simulink subsystem "AS_ExhalationCircuit"  (R2022b)
settings: Solver=VariableStepAuto  StartTime=0.0  StopTime=10.0  RelTol=1e-3
undefined symbols (not defined in the file): cmH2O_to_Pa, Exhalation_Opening_Height, Exhalation_Restrict_Dia, PIDiameter
libraries: fl_lib x6, nesl_utility x3, SimscapeFluids_lib x1
settings Model: DefaultTestHarness=AS_ExhalationCircuit_Harness  Creator=CSN-Simulation  LastModifiedBy=MATLAB
settings DebuggingCC: UnconnectedInputMsg=warning  UnconnectedOutputMsg=warning  UnconnectedLineMsg=warning
settings ModelReferenceCC: EnableRefExpFcnMdlSchedulingChecks=on
settings RTWCC: DLArmComputeVersion=19.05

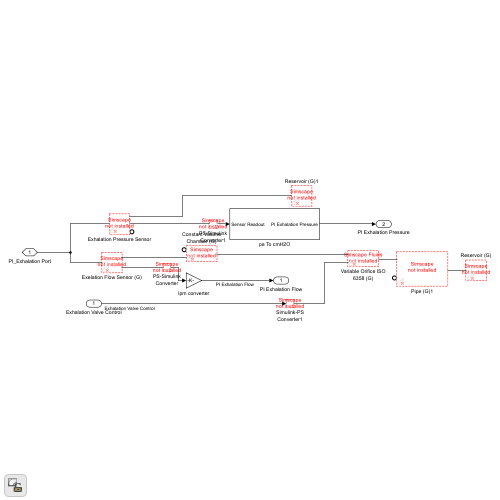
[thumbnail: Simulink's stored preview of the top-level diagram]
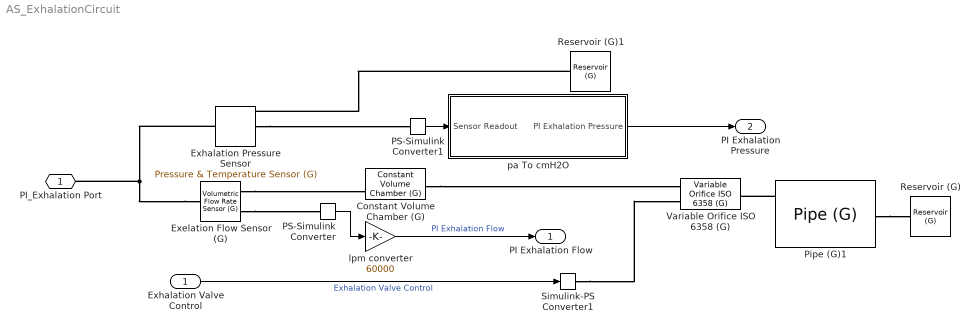
== system AS_ExhalationCircuit ==
  Exhalation Valve Control : Inport
  Constant Volume Chamber (G) : fl_lib/Gas/Elements/Constant Volume Chamber (G)  volume=12000 mm^3  num_ports=foundation.enum.num_ports.two  area_A=pi*(PIDiameter/2)^2 mm^2  area_B=pi*Exhalation_Restrict_Dia*Exhalation_Opening_Height+1 mm^2  area_C=0.01 m^2  area_D=0.01 m^2  p_I_specify=off  p_I_priority=High  p_I=0.101325 MPa  p_I_nominal_specify=off  p_I_nominal_unit=MPa  p_I_nominal_value=1  T_I_specify=off  T_I_priority=High  T_I=293.15 K  T_I_nominal_specify=off  T_I_nominal_unit=K  T_I_nominal_value=1  rho_chamber_specify=off  rho_chamber_priority=None  rho_chamber=1.2 kg/m^3  rho_chamber_nominal_specify=off  rho_chamber_nominal_unit=kg/m^3  rho_chamber_nominal_value=1
      settings: InternalSimscapePortConfiguration="{\"Bottom\":[],\"Left\":[{\"id\":\"A\",\"label\":\"A\",\"type\":\"foundation.gas.gas\"},{\"id\":\"H\",\"label\":\"H\",\"type\":\"foundation.thermal.thermal\"}],\"Right\":[{\"id\":\"B\",\"label\":\"B\",\"type\":\"foundation.gas.gas\"}],\"Top\":[]}"
  Exelation Flow Sensor (G) : fl_lib/Gas/Sensors/Volumetric Flow Rate Sensor (G)
      settings: InternalSimscapePortConfiguration="{\"Bottom\":[],\"Left\":[{\"id\":\"A\",\"label\":\"A\",\"type\":\"foundation.gas.gas\"}],\"Right\":[{\"id\":\"B\",\"label\":\"B\",\"type\":\"foundation.gas.gas\"},{\"id\":\"V\",\"label\":\"V\",\"type\":\"output\"}],\"Top\":[]}"
  Exhalation Pressure Sensor : fl_lib/Gas/Sensors/Pressure & Temperature Sensor (G)
      settings: InternalSimscapePortConfiguration="{\"Bottom\":[],\"Left\":[{\"id\":\"A\",\"label\":\"A\",\"type\":\"foundation.gas.gas\"}],\"Right\":[{\"id\":\"B\",\"label\":\"B\",\"type\":\"foundation.gas.gas\"},{\"id\":\"P\",\"label\":\"P\",\"type\":\"output\"},{\"id\":\"T\",\"label\":\"T\",\"type\":\"output\"}],\"Top\":[]}"
  PS-Simulink Converter : nesl_utility/PS-Simulink Converter  PhysicalDomain=network_engine_domain  SubClassName=ps_output  LeftPortType=input  RightPortType=output  PseudoPeriodic=off  Frequencies=[]  Unit=inherit  AffineConversion=off
  PS-Simulink Converter1 : nesl_utility/PS-Simulink Converter  PhysicalDomain=network_engine_domain  SubClassName=ps_output  LeftPortType=input  RightPortType=output  PseudoPeriodic=off  Frequencies=[]  Unit=inherit  AffineConversion=off
  Pipe (G)1 : fl_lib/Gas/Elements/Pipe (G)  length=5 mm  area=pi*Exhalation_Restrict_Dia*Exhalation_Opening_Height+1 mm^2  Dh=PIDiameter mm  length_add=0.1 m  roughness=15e-6 m  Re_lam=2000  Re_tur=4000  shape_factor=64  Nu_lam=3.66  p_I_specify=off  p_I_priority=High  p_I=0.101325 MPa  p_I_nominal_specify=off  p_I_nominal_unit=MPa  p_I_nominal_value=1  T_I_specify=on  T_I_priority=High  T_I=T_room degC  T_I_nominal_specify=off  T_I_nominal_unit=K  T_I_nominal_value=1  rho_pipe_specify=off  rho_pipe_priority=None  rho_pipe=1.2 kg/m^3  rho_pipe_nominal_specify=off  rho_pipe_nominal_unit=kg/m^3  rho_pipe_nominal_value=1
  Reservoir (G) : fl_lib/Gas/Elements/Reservoir (G)  pressure_spec=foundation.enum.pressure_spec.atmospheric  reservoir_pressure=0.101325 MPa  reservoir_temperature=T_room degC  area_A=pi*(PIDiameter/2)^2 mm^2
  Reservoir (G)1 : fl_lib/Gas/Elements/Reservoir (G)  pressure_spec=foundation.enum.pressure_spec.atmospheric  reservoir_pressure=0.101325 MPa  reservoir_temperature=293.15 K  area_A=0.01 m^2
  Simulink-PS Converter1 : nesl_utility/Simulink-PS Converter  PhysicalDomain=network_engine_domain  SubClassName=ps_input  LeftPortType=input  RightPortType=output  PseudoPeriodic=off  Frequencies=[]  NoiseDistribution=none  NoiseParameters=[]  Unit=1  AffineConversion=off  FilteringAndDerivatives=provide  SimscapeFilterOrder=1  InputFilterTimeConstant=0.001  UdotUserProvided=0
  Variable Orifice ISO 6358 (G) : SimscapeFluids_lib/Gas/Valves & Orifices/Variable Orifice ISO 6358 (G)  iso_cond_spec=fluids.gas.enum.iso_cond_spec.area  iso_opening_spec_C=fluids.gas.enum.iso_opening_spec.linear  C_max=1.6 l/s/bar  C_min=1e-5 l/s/bar  B_crit=0.3  opening_C_TLU=0 : 0.2 : 1  C_TLU=[1e-05, .32, .64, .96, 1.28, 1.6] l/s/bar  B_crit_TLU=0.3 * ones(1, 6)  m=0.5  iso_opening_spec_Cv=fluids.gas.enum.iso_opening_spec.linear  Cv_max=0.4  Cv_min=1e-6  opening_Cv_TLU=0 : 0.2 : 1  Cv_TLU=[1e-06, .08, .16, .24, .32, .4]  iso_opening_spec_Kv=fluids.gas.enum.iso_opening_spec.linear  Kv_max=0.3  Kv_min=1e-6  opening_Kv_TLU=0 : 0.2 : 1  Kv_TLU=[1e-06, .06, .12, .18, .24, .3]  iso_opening_spec_area=fluids.gas.enum.iso_opening_spec.linear  restriction_area_max=pi*Exhalation_Restrict_Dia*Exhalation_Opening_Height mm^2  restriction_area_min=1e-10 mm^2  opening_area_TLU=0 : 0.2 : 1  restriction_area_TLU=[1e-10, 2e-06, 4e-06, 6e-06, 8e-06, 1e-05] m^2  area=pi*Exhalation_Restrict_Dia*Exhalation_Opening_Height+1 mm^2  B_lam=0.999  T0=293.15 K  rho0=1.185 kg/m^3  smoothing_factor=0
      settings: InternalSimscapePortConfiguration="{\"Bottom\":[],\"Left\":[{\"id\":\"A\",\"label\":\"A\",\"type\":\"foundation.gas.gas\"},{\"id\":\"L\",\"label\":\"L\",\"type\":\"input\"}],\"Right\":[{\"id\":\"B\",\"label\":\"B\",\"type\":\"foundation.gas.gas\"}],\"Top\":[]}"
  lpm converter : Gain  Gain=60000
  pa To cmH2O : Subsystem
  PI_Exhalation Port : PMIOPort  Side=Left
  PI Exhalation Flow : Outport
  PI Exhalation Pressure : Outport  Port=2
  wires:
  PS-Simulink Converter/1 -> lpm converter/1
  Exhalation Valve Control/1 -> Simulink-PS Converter1/1  "Exhalation Valve Control"
  lpm converter/1 -> PI Exhalation Flow/1  "PI Exhalation Flow"
  PS-Simulink Converter1/1 -> pa To cmH2O/1(Sensor Readout)
  pa To cmH2O/1(PI Exhalation Pressure) -> PI Exhalation Pressure/1
  connections:
  Exelation Flow Sensor (G)/LConn1 -- PI_Exhalation Port/RConn1 -- Exhalation Pressure Sensor/LConn1
  Constant Volume Chamber (G)/RConn1 -- Variable Orifice ISO 6358 (G)/LConn1
  Pipe (G)1/LConn1 -- Variable Orifice ISO 6358 (G)/RConn1
  Exelation Flow Sensor (G)/RConn1 -- Constant Volume Chamber (G)/LConn1
  Pipe (G)1/RConn1 -- Reservoir (G)/LConn1
  Exhalation Pressure Sensor/RConn2 -- PS-Simulink Converter1/LConn1
  Exelation Flow Sensor (G)/RConn2 -- PS-Simulink Converter/LConn1
  Reservoir (G)1/LConn1 -- Exhalation Pressure Sensor/RConn1
  Simulink-PS Converter1/RConn1 -- Variable Orifice ISO 6358 (G)/LConn2

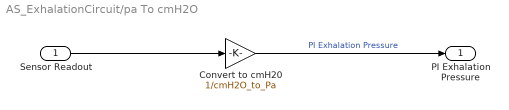
== system AS_ExhalationCircuit/pa To cmH2O ==
  Sensor Readout : Inport
  Convert to cmH20 : Gain  Gain=1/cmH2O_to_Pa
  PI Exhalation Pressure : Outport
  wires:
  Convert to cmH20/1 -> PI Exhalation Pressure/1  "PI Exhalation Pressure"
  Sensor Readout/1 -> Convert to cmH20/1
